simulink model "walkingRobotCapture2"  (R2020a)
settings: Solver=ode15s  StartTime=0.0  StopTime=inf  EnableMultiTasking=on
PreLoadFcn:
  | % run script to load up the parameters
  | robotParameters
values from neighbouring files (symbols this model uses):
  foot_x = 0.17    [robotParameters.m]
  foot_y = 0.17    [robotParameters.m]
  foot_z = 0.02    [robotParameters.m]
  init_angs_L = zeros(6,1)    [robotParameters.m]
  init_angs_R = zeros(6,1)    [robotParameters.m]
  leg_width = 0.08    [robotParameters.m]
  lower_leg_length = 0.38    [robotParameters.m]
  plane_x = 3    [robotParameters.m]    (also in startupWalkingRobot.m = 30)
  plane_y = 50    [robotParameters.m]
  plane_z = height_plane    (= 0.025)    [robotParameters.m]
  s = Rp(:,2)    [invKinBody2Foot.m]
  torso_height = 0.35    [robotParameters.m]
  torso_length = 0.20    (= 0.2)    [robotParameters.m]
  torso_offset_height = 0    [robotParameters.m]
  torso_offset_length = 0    [robotParameters.m]
  torso_width = 0.24    [robotParameters.m]
  Ts = 0.005    [startupWalkingRobot.m]
  upper_leg_length = 0.40    (= 0.4)    [robotParameters.m]
  X = mat(1,4)    [Transform.m]
  Y = mat(2,4)    [Transform.m]
  Z = mat(3,4)    [Transform.m]
libraries: sm_lib x57, walkingRobotUtils x17, nesl_utility x4, simulink x1
(part 3 of 3)

== stateflow chart walkingRobotCapture2/Chart ==
  state StandBy
    entry:
    idxmax = 0.5/TS;
    during:
    idx = idx + 1;
  note: Constants
      | Multiple Constants are used in this chart. Most constants are CAPITALIZED.
      | TS: sample time of trajectory
      | W: sqrt(g/zModel)
      | STEPTIME: duration of a single step
      | AD,BD, CD, DD: discrete state space representation of LIPM
      |
      | ZMODEL: the height of pendulum model; this is the height at which robot will walk
      | RWDITH: the width of the robot
      | RHEIGHT: the height of the robot when standing straigh
      |
      | TB_FR: the transform matrix from body to right foot at bend-knee position
      | TB_FL: the transfom matrix from body to left foot at bend-knee position
  note: Local Data
      | Multiple local variables are used in this chart. They are used in muliple area
      | Tw_b: transform matrix from world to body
  state BendKnee
    entry:
    endPoseRight =           [0 -1 0 RWIDTH/2;0 0 1 0;-1 0 0 -RHEIGHT;0 0 0 1];
    endPoseRightTarget = TB_FR;
    endPoseLeft =          [0 -1 0 -RWIDTH/2;0 0 1 0;-1 0 0 -RHEIGHT;0 0 0 1];
    endPoseLeftTarget = TB_FL;
    tduration = 1.5;
    xyzqtrajr = getTrajectory(endPoseRight, endPoseRightTarget, tduration);
    xyzqtrajl = getTrajectory(endPoseLeft, endPoseLeftTarget, tduration);
    idx = 1; idxmax = round(tduration/TS);
    endPoseRight = vec2Tform(xyzqtrajr(:,idx));
    endPoseLeft = vec2Tform(xyzqtrajl(:,idx));
    idx = idx + 1;
    during:
    endPoseRight = vec2Tform(xyzqtrajr(:,idx));
    endPoseLeft = vec2Tform(xyzqtrajl(:,idx));
    idx = idx + 1;
  state RightStance
    entry:
    getWalkingTrajectory(RIGHTMODE);
    during:
    %endPoseRight = xyzq2Tform(stanceXyzq(:,idx));
    endPoseRight = TTc_pf(1:4,1:4,idx);
    endPoseLeft = xyzq2Tform(swingXyzq(:,idx));
    idx = idx + 1;
  state LeftStance
    entry:
    getWalkingTrajectory(LEFTMODE);
    during:
    %endPoseLeft = xyzq2Tform(stanceXyzq(:,idx));
    endPoseLeft = TTc_pf(1:4,1:4,idx);
    endPoseRight = xyzq2Tform(swingXyzq(:,idx));
    idx = idx + 1;
  state WalkReady
    entry:
    endPoseRight = endPoseRightTarget;
    endPoseLeft = endPoseLeftTarget;
    endPoseRightTarget(1:3,4) = [0.0; 0.0; -ZMODEL];
    endPoseLeftTarget(1:3,4) = [-0.24; 0.0; -ZMODEL];
    tduration = 1.5;
    xyzqtrajr = getTrajectory(endPoseRight, endPoseRightTarget, tduration);
    xyzqtrajl = getTrajectory(endPoseLeft, endPoseLeftTarget, tduration);
    idxmax = round(tduration/TS);
    endPoseRight = vec2Tform(xyzqtrajr(:,idx));
    endPoseLeft = vec2Tform(xyzqtrajl(:,idx));
    idx = idx + 1;
    during:
    endPoseRight = vec2Tform(xyzqtrajr(:,idx));
    endPoseLeft = vec2Tform(xyzqtrajl(:,idx));
    idx = idx + 1;
  (default) -> StandBy : {idx = 1;}
  StandBy -> BendKnee : [idx > idxmax]
      | {idx = 1;}
  RightStance -> LeftStance : [idx > idxmax]{idx = 1;}
  BendKnee -> WalkReady : [idx > idxmax]
      | {idx = 1;}
  LeftStance -> RightStance : [idx > idxmax]{idx = 1;}
  WalkReady -> RightStance : [idx > idxmax]
      | {idx = 1;}
  data: whichStance function_input; currMat function_input; targetMat function_input; taction function_input; xyzqtrajectory function_output; xyzqtrajectory function_output; currMat function_input; targetMat function_input; xyzqtrajectory function_output; currMat function_input; targetMat function_input; TS constant double =Ts; ZMODEL constant double =zModel; RWIDTH constant double =torso_width; RHEIGHT constant double =init_height; endPoseLeftTarget local size=[4,4]; endPoseRightTarget local size=[4,4]; endPoseRight output size=[4,4] =[0 -1 0 0.12;0 0 1 0;-1 0 0 -0.78;0 0 0 1]; endPoseLeft output size=[4,4] =[0 -1 0 -0.12;0 0 1 0;-1 0 0 -0.78;0 0 0 1]; xyzqtrajr local size=[7, 2500]; xyzqtrajl local size=[7, 2500]; tduration local; idxmax local; idx local; RIGHTMODE constant double =1; LEFTMODE constant double =2; deltaPos input size=2; deltaYaw input; TB_FR constant double size=[4,4] =[0 -1 0 torso_width/2;0 0 1 0;-1 0 0 -zModel;0 0 0 1];; TB_FL constant double size=[4,4] =[0 -1 0 -torso_width/2;0 0 1 0;-1 0 0 -zModel;0 0 0 1];; W constant double =w; STEPTIME constant double =desiredStepTime; Tw_b local =[1 0 0 0;0 1 0 0;0 0 1 zModel;0 0 0 1]; AD constant double size=[4, 4] =Ad; BD constant double size=[4,2] =Bd; CD constant double size=[2,4] =Cd; DD constant double size=[2,2] =Dd; state0 local =[x0 dx0 y0 dy0]'; state1 local =zeros(4,1); meas1 local =zeros(2,1); u0 local =zeros(2,1); Tc_pf local size=[4,4,2500]; SWINGHEIGHT constant double =0.1; measurementvec local =zeros(3,250); Tw_c local =[1 0 0 0;0 1 0 0;0 0 1 0;0 0 0 1]; Tw_c1 local =[1 0 0 0;0 1 0 0;0 0 1 0;0 0 0 1]; swingXyzq local size=[7,2500]; stanceXyzq local size=[7,2500]; TTc_pf local size=[4,4,2500]
  function getWalkingTrajectory(whichStance):
    | function getWalkingTrajectory(whichStance)
    | % Tb, Tb1: The "capture-point body pose" is an capture-point body pose I keep track of to determine
    | % capture point. This is not really where the actual body of the robot will
    | % be, rather this is some pose that the robot will be around at during the middle
    | % of its stance trajectory. capture-point body pose is essentially something that helps
    | % me get the desired end-of-step capture point based on input. Remember the
    | % key input for this algorithm is the capture point. In the end I just want
    | % some capture point to work with. This capture-point body pose keep track of
    | % the input to give me that capture point. 
    | % The actual body of the robot is described with c Tc, Tw_c (center of
    | % body)
    | 
    | % transform from current capture-point body pose to next end of step capture-point 
    | % body pose
    | Tb_b1 = eye(4); 
    | Tb_b1(1,1) =  cos(deltaYaw); Tb_b1(1,2) = sin(deltaYaw);
    | Tb_b1(2,1) = -sin(deltaYaw); Tb_b1(2,2) = cos(deltaYaw);
    | Tb_b1(1,4) = deltaPos(1); 
    | Tb_b1(2,4) = deltaPos(2); 
    | 
    | % transform from body to foot's default (standing) pose
    | if whichStance == 1 % right stance 
    |     Tf = TB_FR; 
    |     Tstance = TB_FR; 
    |     Tswing  = TB_FL; 
    | else % == 2 left stance 
    |     Tf = TB_FL;  
    |     Tstance = TB_FL; 
    |     Tswing = TB_FR; 
    | end
    | 
    | % Tw_b:   transform from world to capture-point body 
    | % Tw_b1:  transform from world to capture-point body at end of step
    | % Tw_sf : transform from world to swing foot at beginning of step 
    | %         This swing foot just took off, it will go to Tw_sf1 at the end of
    | %         the step 
    | % Tw_sfl: transform from world to swing foot at end of step 
    | %         this is the next step's plant foot 
    | %         this is where the swing foot should land on 
    | %         this is based on desired capture point (thus input) 
    | % Tw_pf : transform from world to plant foot at beginning of step
    | Tw_b1  = Tw_b  * Tb_b1;
    | Tw_sf1 = Tw_b1 * Tswing;
    | 
    | % based on current capture point cx, cy and desired capture point 
    | % (which is where you will put your next stance foot down) at the
    | % end of step (cxeos, cyeos), calculate the pendulum base (ZMP) px and py. 
    | cxeos = Tw_sf1(1,4)
    | cyeos = Tw_sf1(2,4) 
    | cx = state0(1) + state0(2)/W % current capture point x
    | cy = state0(3) + state0(4)/W % current capture point y 
    | px = findZMP(W, STEPTIME, cxeos, cx); 
    | py = findZMP(W, STEPTIME, cyeos, cy); 
    | u0 = [px; py]
    | 
    | % simulate the pendulum to get the trajectory out of it; 
    | % the ZMP (px, py) is the base of pendulum 
    | % This calculates the trajectory of robot's ACTUAL body w.r.t. world. Since
    | % this only calculates the x and y trajectory of it
    | idxmax = round(STEPTIME/TS); 
    | state0
    | simulateLipm();
    | state0
    | Tw_c(1:3,4) = measurementvec(1:3,1);
    | Tw_c1(1:3,4) = measurementvec(1:3,idxmax); 
    | Tw_c1(1:3,1:3) = Tw_b1(1:3,1:3);
    | Tw_c
    | Tw_c1
    | 
    | % Get the swing foot based on Tw_c
    | % swing foot beginning is basically where the plant(stance) foot was at the
    | % end of last step
    | if whichStance == 1 % right stance
    |     Tc_sf = endPoseLeft;
    | else % left stance
    |     Tc_sf = endPoseRight;
    | end 
    | Tc1_sf1 = TransformInverse(Tw_c1) * Tw_sf1;
    | 
    | % get the swing foot trajectory 
    | swingXyzq = generateSwingTraj(Tc_sf, Tc1_sf1);
    | 
    | % Tpf_c : transform from plant foot to actual center of body 
    | %         note Tb was reserved for the capture-point body that keep track of
    | %         user input 
    | % Based on plant foot and body x,y trajectory w.r.t. world, calculate the 
    | % pose + orientation trajectory w.r.t. plant foot Tpf_c
    | % then get Tc_pf
    | % Tw_pf : plant foot is found earlier from findZMP
    | Tw_pf = Tstance; 
    | Tw_pf(1:3,4) = [px; py; 0]; 
    | Tpf_w = TransformInverse(Tw_pf); 
    | Tpf_c = Tpf_w * Tw_c; 
    | Tpf_c1 = Tpf_w * Tw_c1; 
    | % Tpf_c = zeros(4,4,idxmax); 
    | % Tpf_c(4,4,:) = 1; 
    | % % Tpf_c = [0 -1 0;0 0 1;-1 0 0]
    | % Tpf_c(1,2,:) = -1;
    | % Tpf_c(2,3,:) =  1;
    | % Tpf_c(3,1,:) = -1;
    | % Tpf_c(1:3,1:idxmax) = measurementvec(1:3,1:idxmax); 
    | Tc_pf = TransformInverse(Tpf_c);
    | Tc1_pf = TransformInverse(Tpf_c1); 
    | stanceXyzq = generateXyzqTraj(Tc_pf, Tc1_pf); 
    | % TODO: transform measurementvec from world coordinate to 
    | % body_pf coordinate 
    | TTw_c = zeros(4,4,idxmax); 
    | TTw_c(4,4,:) = 1; 
    | TTw_c(1:3,1:3,1:idxmax) = rottraj(Tw_c(1:3,1:3),Tw_c1(1:3,1:3), [0 STEPTIME], 0:TS:STEPTIME-TS);
    | % is measurementvec Tw_c? 
    | for i = 1:idxmax
    |     TTw_c(1:2,4,i) = measurementvec(1:2,i); 
    | end 
    | % get the inverse 
    | TTc_w = zeros(size(TTw_c)); 
    | for i = 1:idxmax
    |     TTc_w(:,:,i) = TransformInverse(TTw_c(:,:,i)); 
    | end 
    | 
    | TTc_pf = zeros(4,4,idxmax); 
    | for i = 1:idxmax
    |     TTc_pf(:,:,i) = TTc_w(:,:,idx) * Tw_pf; 
    | end 
    | 
    | Pw = zeros(4,idxmax);
    | Pw(4,:) = 1; 
    | Pw(3,:) = ZMODEL; 
    | Pw(1:2,1:idxmax) = measurementvec(1:2,1:idxmax); 
    | Ppf = Tpf_w * Pw; 
    | stanceXyzq(1:3,1:idxmax) = Ppf(1:3,1:idxmax);
    | 
    | % update the pose of capture-point of the robot
    | Tw_b = Tw_b1;
    | % update the pose of actual center of body 
    | Tw_c = Tw_c1; 
    | 
    | % % Tw_b: transform from world to body 
    | % % Tw_b1: transform from world to body at end of step
    | % % Tw_f: transform from world to foot 
    | % % Tb_fl: ''       from body to foot left
    | % Tw_fr0 = Tw_b * TB_FR; % currrent world to right foot transform 
    | % Tw_b   = Tw_b * Tb_bp; % next step world to body 
    | % Tw_fr1 = Tw_b * TB_FR; % next world to right foot transform 
    | % Tw_fl  = Tw_b * TB_FL;
    | % % Tb_fl = Tb_bp * TB_FL; 
    | % Tb_fr1 = Tb_bp * TB_FR; % end of step body to right foot transform 
    | % 
    | % % based on current capture point cx, cy and desired capture point at the
    | % % end of step (cxeos, cyeos), calculate the needed stance foot location (ZMP)
    | % % px and py. 
    | % cxeos  = Tw_fl(1,4);
    | % cyeos  = Tw_fl(2,4);
    | % [cx, cy] = getCapturePoint(state0,W);
    | % [px, py] = findZMP(cx, cy, W, STEPTIME, cxeos, cyeos);
    | % u0 = [px py]';
    | % fholdx = cx;
    | % fholdy = cy;
    | % Tw_fr1(1,4) = fholdx; Tw_fr1(2,4) = fholdy; 
    | % 
    | % % the LIPM trajectory based on px, py (u0) will get you to where you want
    | % % at the end of step 
    | % idxmax = round(STEPTIME/TS);
    | % [measvec, state1] = simulateLipm(state0, u0, idxmax);
    | % state0 = state1;
    | % % get world to new body pose based on state
    | % Tw_bp = Tw_b;
    | % Tw_bp(1,4) = state1(1); Tw_bp(2,4) = state1(3); 
    | % % Get inverse
    | % Tbp_w = eye(4);
    | % Tbp_w(1:3,1:3) = Tw_bp(1:3,1:3)'; 
    | % Tbp_w(1:3,4) = -Tw_bp(1:3,1:3)'*Tw_bp(1:3,4); 
    | % Tbp_fl = Tbp_w * Tw_fl; 
    | % 
    | % % now translate those points into what robot can understand. Get the points
    | % % w.r.t. the robot 
    | % endPoseLeftTarget(1:3,1:3) = TB_FL(1:3,1:3); 
    | % Tw_b(1,4) = state1(1); Tw_b(2,4) = state1(3); 
    | % Tb_w = TransformInverse(Tw_b); 
    | % Tb_fl = Tb_w * Tw_fl; 
    | % endPoseLeftTarget(1,4) = Tb_fl(1,4); %cxeos - state1(1);
    | % endPoseLeftTarget(2,4) = Tb_fl(2,4); %cyeos - state1(3);
    | % % tformtrajl = generateSwingTraj2(endPoseLeft, endPoseLeftTarget); 
    | % xyzqtrajl = generateSwingTraj(endPoseLeft, endPoseLeftTarget);
    | % % stancetraj = getStanceTraj(measvec,fholdx,fholdy);
    | % 
    | % % only orientation will be used from target matrix 
    | % % TODO: change getStanceTraj2 to only take 3x3 rotation matrix 
    | % % Stance foot will rotate the body to desired orientation end of step 
    | % endPoseRightTarget(1:3, 1:3) = Tb_fr1(1:3, 1:3); 
    | % xyzqtrajr = getStanceTrajectory(endPoseRight, endPoseRightTarget, ...
    | %                            measvec, Tw_fr0, STEPTIME, TS);
    | % % xyzqtrajr = getStanceTraj2(endPoseRight, endPoseRightTarget, ...
    | % %                            measvec, fholdx, fholdy);
    | % xyzqtrajr
    | 
    | end
  function simulateLipm:
    | function simulateLipm
    | % remember that in Stateflow, all variables are pretty much global
    | % variables
    |     measurementvec(3,:) = ZMODEL; 
    |     
    |     meas1 = CD*state0 + DD*u0;
    |     measurementvec(1:2,1) = meas1;
    |     for temp = 2:idxmax 
    |         state1 = AD*state0 + BD*u0;
    |         meas1  = CD*state1 + DD*u0;
    |         measurementvec(1:2,temp) = meas1;
    |         state0 = state1;
    |     end
    | end
  function xyzqtrajectory = getTrajectory(currMat, targetMat, taction):
    | function xyzqtrajectory = getTrajectory(currMat, targetMat, taction)
    | 
    | quat = quaternion(currMat(1:3,1:3), 'rotmat', 'frame'); 
    | quat = quat.compact; 
    | quattarget = quaternion(targetMat(1:3,1:3), 'rotmat', 'frame');
    | quattarget = quattarget.compact; 
    | 
    | x = currMat(1,4); y = currMat(2,4); z = currMat(3,4); 
    | xt = targetMat(1,4); yt = targetMat(2,4); zt = targetMat(3,4); 
    | 
    | currPts = [x y z quat]';
    | targetPts = [xt yt zt quattarget]'; 
    | 
    | wpts = [currPts targetPts]; 
    | tpts = [0 taction];
    | tvec = 0:TS:taction; 
    | 
    | [xyzqtrajectory, ~, ~, ~] = cubicpolytraj(wpts, tpts, tvec);
  function xyzqtrajectory = generateSwingTraj(currMat, targetMat):
    | function xyzqtrajectory = generateSwingTraj(currMat, targetMat)
    | 
    | quat = quaternion(currMat(1:3,1:3), 'rotmat', 'frame'); 
    | quat = quat.compact; 
    | quattarget = quaternion(targetMat(1:3,1:3), 'rotmat', 'frame');
    | quattarget = quattarget.compact; 
    | 
    | x0 = currMat(1,4);     y0 = currMat(2,4);     z0 = currMat(3,4); 
    | x2 = targetMat(1,4);   y2 = targetMat(2,4);   z2 = targetMat(3,4); 
    | x1 = (x0 + x2)/2;      y1 = (y0 + y2)/2;      z1 = z0 + SWINGHEIGHT; 
    | 
    | pts0 = [x0 y0 z0 quat]';
    | pts1 = [x1 y1 z1 quattarget]'; 
    | pts2 = [x2 y2 z2 quattarget]'; 
    | 
    | wpts = [pts0 pts1 pts2]; 
    | tpts = [0 STEPTIME/2 STEPTIME];
    | tvec = 0:TS:STEPTIME; 
    | 
    | [xyzqtrajectory, ~, ~, ~] = cubicpolytraj(wpts, tpts, tvec); 
    | end
  function xyzqtrajectory = generateXyzqTraj(currMat, targetMat):
    | function xyzqtrajectory = generateXyzqTraj(currMat, targetMat)
    | 
    | quat = quaternion(currMat(1:3,1:3), 'rotmat', 'frame'); 
    | quat = quat.compact; 
    | quattarget = quaternion(targetMat(1:3,1:3), 'rotmat', 'frame');
    | quattarget = quattarget.compact; 
    | 
    | x0 = currMat(1,4);     y0 = currMat(2,4);     z0 = currMat(3,4); 
    | x2 = targetMat(1,4);   y2 = targetMat(2,4);   z2 = targetMat(3,4); 
    | x1 = (x0 + x2)/2;      y1 = (y0 + y2)/2;      z1 = (z0 + z2)/2; 
    | 
    | pts0 = [x0 y0 z0 quat]';
    | pts1 = [x1 y1 z1 quattarget]'; 
    | pts2 = [x2 y2 z2 quattarget]'; 
    | 
    | wpts = [pts0 pts1 pts2]; 
    | tpts = [0 STEPTIME/2 STEPTIME];
    | tvec = 0:TS:STEPTIME; 
    | 
    | [xyzqtrajectory, ~, ~, ~] = cubicpolytraj(wpts, tpts, tvec); 
    | end
